simulink model "assignment3"  (R2017b)
settings: Solver=VariableStepAuto  StartTime=0.0  StopTime=10.0  RelTol=1e-3
settings Model: Creator=Raymond  LastModifiedBy=Raymond

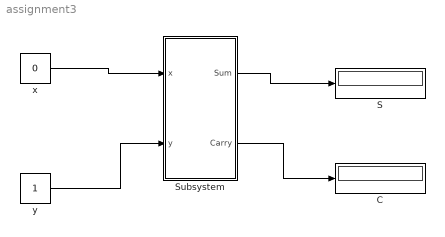
== system assignment3 ==
  C : Display
  S : Display
  Subsystem : Subsystem
  x : Constant  Value=0  OutDataTypeStr=boolean
  y : Constant  OutDataTypeStr=boolean
  wires:
  x/1 -> Subsystem/1(x)
  y/1 -> Subsystem/2(y)
  Subsystem/1(Sum) -> S/1
  Subsystem/2(Carry) -> C/1

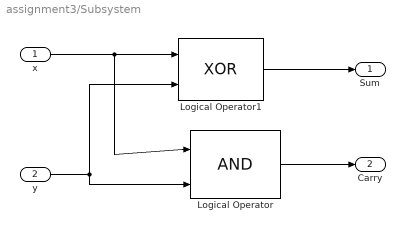
== system assignment3/Subsystem ==
  x : Inport
  y : Inport  Port=2
  Logical Operator : Logic  IconShape=distinctive  AllPortsSameDT=off  OutDataTypeStr=boolean
  Logical Operator1 : Logic  Operator=XOR  IconShape=distinctive  AllPortsSameDT=off  OutDataTypeStr=boolean
  Sum : Outport
  Carry : Outport  Port=2
  wires:
  x/1 -> Logical Operator/1, Logical Operator1/1
  y/1 -> Logical Operator1/2, Logical Operator/2
  Logical Operator/1 -> Carry/1
  Logical Operator1/1 -> Sum/1
